simulink library "Simple_lib"  (R2018b)
settings: Solver=ode45  StartTime=0.0  StopTime=10.0  RelTol=1e-3  EnableMultiTasking=on
undefined symbols (not defined in the file or in its folder): Acceptance, beta, C, C_J, C_P, c_wall, dGain, DiscIntNeverNeededParam, Duplex, Electrical_lib, grab, h_fe, i, i3, K_T, Kman, KmanCE, mu_s, n_rev, R_arm, Simplex, systemTs, tau_0, TinIC, Ts, w_0, wallMass, Watch_lib
libraries: $bdroot x407, PlantUtilityBlockset_lib x30, peGeneralControl x22, simulink x11
(part 4 of 14)

== system Simple_lib/Magnetic ==
  BiGain : Subsystem  mask{k_level=-1, k_flow=-1}
      mask prompts: k_level "Level Gain"; k_flow "Flow Gain"
      settings: AttributesFormatString="%<k_flow>   %<k_level>"
      mask Display:
      | patch( [0 1 0],[1 0 -1])
      | plot( [0 -1 0],[1 0 -1])
  Core : Subsystem  mask{b=.5}
      mask prompts: b "Damping coefficient (Ns/m)"
      settings: AttributesFormatString=%<b> Ns/m
      mask Display:
      | plot([-1 1], [0.5 0.5])
      | plot([-1 1], [-0.5 -0.5])
      | 
      | color('white')
      | plot([-1 1 1 -1 -1], [-1 -1 1 1 -1])
  Core_old : Subsystem  mask{b=.9*sqrt(2e-1*3e-1)}
      mask prompts: b "Damping coefficient (Ns/m)"
      settings: AttributesFormatString=%<b> Ns/m
      mask Display:
      | plot([-1 1], [0.5 0.5])
      | plot([-1 1], [-0.5 -0.5])
      | 
      | color('white')
      | plot([-1 1 1 -1 -1], [-1 -1 1 1 -1])
  Friction : Subsystem  mask{grab=1, s=1, Ki=100}
      mask prompts: s "sigma"
      mask Display:
      | plot([0 .1],[1.7 1.7]);
      | plot([0 .1],[-1.7 -1.7]);
      | plot([.2 .3],[1.7 1.7]);
      | plot([.2 .3],[-1.7 -1.7]);
      | plot([.4 .5],[1.7 1.7]);
      | plot([.4 .5],[-1.7 -1.7]);
      | plot([.6 .7],[1.7 1.7]);
      | plot([.6 .7],[-1.7 -1.7]);
      | plot([.8 .9],[1.7 1.7]);
      | plot([.8 .9],[-1.7 -1.7]);
      | 
      | patch([0 1 1 0],[2 2 2.1 2.1]);
      | patch([0 1 1 0],[-2 -2 -2.1 -2.1]);
      | color('white');
      | plot([0 1],[3 3]);
      | plot([0 1],[-3 -3]);
  Sink : Subsystem  mask{m=0.01}
      mask prompts: m "Inertia (kg)"
      settings: AttributesFormatString=%<m> kg
      mask Display:
      | %color('white');
      | %plot([0 4],[1 1]);
      | %plot([0 4],[-1 -1]);
      | %color('black')
      | %plot([0 2],[0 0]);
      | plot([-1 -.9 -.8 0 .8 .9 1  .9  .8  0 -.8 -.9 -1],      [ 0  .9 .9 1 .9 .9 0 -.9 -.9 -1 -.9 -.9  0]);
  Source : Subsystem  mask{m=0.1, v_0=0}
      mask prompts: m "Inertia (kg)"; v_0 "Initial velocity (m/s)"
      settings: AttributesFormatString=%<m> kg
      mask Display:
      | %color('white');
      | %plot([-1 4],[1 1]);
      | %plot([-1 4],[-1 -1]);
      | %color('black')
      | %plot([1 4],[0 0]);
      | plot([-1 -.9 -.8 0 .8 .9 1  .9  .8  0 -.8 -.9 -1],      [ 0  .9 .9 1 .9 .9 0 -.9 -.9 -1 -.9 -.9  0]);
      | %plot([4 4.5 4.5 4],[0 -0.25 0.25 0])
  SpringDamper : Subsystem  mask{k_spring=1000, b_damper=0, b_spring=inf, m_out=0, m_split=0, v_0=0, s_0=0}
      mask prompts: k_spring "Stiffness (N/m)"; b_damper "Parallel Damping (Ns/m)"; b_spring "Series Damping (Ns/m)"; m_out "Output Inertia (kg)"; m_split "Split inertia (kg)"; v_0 "Initial speed (m/s)"; s_0 "Initial rotation (m)"
      mask Display:
      | %color('white')
      | %plot([-1 1 1 -1 -1], [-1 -1 1 1 -1])
      | %color('black')
      | %plot([1.0 1.18 1.18 1.0], [0 .2 -.2 0])
      | plot(-1+2*[-0.0625
      |    -0.0421
      |    -0.0129
      |     0.0230
      |     0.0625
      |     0.1020
      |     0.1379
      |     0.1671
      |     0.1875
      |     0.1984
      |     0.2004
      |     0.1958
      |     0.1875
      |     0.1792
      |     0.1746
      |     0.1766
      |     0.1875
      |     0.2079
      |     0.2371
      |     0.2730
      |     0.3125
      |     0.3520
      |     0.3879
      |     0.4171
      |     0.4375
      |     0.4484
      |     0.4504
      |     0.4458
      |     0.4375
      |     0.4292
      |     0.4246
      |     0.4266
      |     0.4375
      |     0.4579
      |     0.4871
      |     0.5230
      |     0.5625
      |     0.6020
      |     0.6379
      |     0.6671
      |     0.6875
      |     0.6984
      |     0.7004
      |     0.6958
      |     0.6875
      |     0.6792
      |     0.6746
      |     0.6766
      |     0.6875
      |     0.7079
      |     0.7371
      |     0.7730
      |     0.8125
      |     0.8520
      |     0.8879
      |     0.9171
      |     0.9375
      |     0.9484
      |     0.9504
      |     0.9458
      |     0.9375
      |     0.9292
      |     0.9246
      |     0.9266
      |     0.9375], [    0
      |     0.3827
      |     0.7071
      |     0.9239
      |     1.0000
      |     0.9239
      |     0.7071
      |     0.3827
      |     0.0000
      |    -0.3827
      |    -0.7071
      |    -0.9239
      |    -1.0000
      |    -0.9239
      |    -0.7071
      |    -0.3827
      |    -0.0000
      |     0.3827
      |     0.7071
      |     0.9239
      |     1.0000
      |     0.9239
      |     0.7071
      |     0.3827
      |     0.0000
      |    -0.3827
      |    -0.7071
      |    -0.9239
      |    -1.0000
      |    -0.9239
      |    -0.7071
      |    -0.3827
      |    -0.0000
      |     0.3827
      |     0.7071
      |     0.9239
      |     1.0000
      |     0.9239
      |     0.7071
      |     0.3827
      |     0.0000
      |    -0.3827
      |    -0.7071
      |    -0.9239
      |    -1.0000
      |    -0.9239
      |    -0.7071
      |    -0.3827
      |    -0.0000
      |     0.3827
      |     0.7071
      |     0.9239
      |     1.0000
      |     0.9239
      |     0.7071
      |     0.3827
      |     0.0000
      |    -0.3827
      |    -0.7071
      |    -0.9239
      |    -1.0000
      |    -0.9239
      |    -0.7071
      |    -0.3827
      |    -0.0000])
      | 
      | %color('black')
      | plot( [-1 0.3], [0 0]-3 )
      | plot( .3*[1 1],.9*[-1 1]-3 )
      | plot(  [0 1 1 0], [1 1 -1 -1]-3 )
      | %color('white')
      | %plot([-1 1], [1.1 1.1])
      | %plot([-1 1 1 -1 -1], [-1 -1 1 1 -1])
  Stiffness : Subsystem  mask{k_spring=1000, s_0=0, I_spring=0, b_series=inf}
      mask prompts: k_spring "Stiffness (N/m)"; s_0 "Initial displacement (m)"; I_spring "Inertia (kg)"; b_series "Series damping (Ns/m)"
      settings: AttributesFormatString=|
      | %<k_spring> N/m
      | %<s_0> m
      mask Display:
      | %color('black')
      | plot(   [    0     0.3827     0.7071     0.9239     1.0000     0.9239     0.7071     0.3827     0.0000    -0.3827    -0.7071    -0.9239    -1.0000    -0.9239    -0.7071    -0.3827    -0.0000     0.3827     0.7071     0.9239     1.0000     0.9239     0.7071     0.3827     0.0000    -0.3827    -0.7071    -0.9239    -1.0000    -0.9239    -0.7071    -0.3827    -0.0000     0.3827     0.7071     0.9239     1.0000     0.9239     0.7071     0.3827     0.0000    -0.3827    -0.7071    -0.9239    -1.0000    -0.9239    -0.7071    -0.3827    -0.0000     0.3827     0.7071     0.9239     1.0000     0.9239     0.7071     0.3827     0.0000    -0.3827    -0.7071    -0.9239    -1.0000    -0.9239    -0.7071    -0.3827    -0.0000],   -.5+[-0.0625    -0.0421    -0.0129     0.0230     0.0625     0.1020     0.1379     0.1671     0.1875     0.1984     0.2004     0.1958     0.1875     0.1792     0.1746     0.1766     0.1875     0.2079     0.2371     0.2730     0.3125     0.3520     0.3879     0.4171     0.4375     0.4484     0.4504     0.4458     0.4375     0.4292     0.4246     0.4266     0.4375     0.4579     0.4871     0.5230     0.5625     0.6020     0.6379     0.6671     0.6875     0.6984     0.7004     0.6958     0.6875     0.6792     0.6746     0.6766     0.6875     0.7079     0.7371     0.7730     0.8125     0.8520     0.8879     0.9171     0.9375     0.9484     0.9504     0.9458     0.9375     0.9292     0.9246     0.9266     0.9375])
      | color('white')
      | plot([-1 1 1 -1 -1], [-1 -1 1 1 -1])
  _in : Subsystem  InitFcn=""  mask{Level=MMF, Flow=Phi}
      mask prompts: Level "Level variable name:"; Flow "Flow variable name:"
      mask init:
      | init_in
      mask Display:
      | %% Icon for flow in
      | % Signally design
      | %plot([0 2 2 3], [1 1 0 0])
      | %plot([1 3 2 1 0 2], [0.6 0.6 0.4 0.6 0.4 0.4])
      | %patch([1 3 2],[0.6 0.6 0.4])
      | %plot([0 1 1], [1 1 0.6])
      | %plot([1 1 0], [0.4 -1 -1])
      | 
      | %color('white')
      | %plot([0 3], [2 2])
      | %plot([0 3], [-2 -2])
      | 
      | %% Bolder design
      | %patch( [0 1 -1], [0 1 1])
      | %plot( [-1 1], [1.051 1.05])
      | %patch( [-0.1 -0.1 -1], [0.95 0 0.95])
      | patch( [-0.1 -0.1 -1], [1 0 1])
      | patch( [0.1 0.1 1], [1 0 1])
      | plot( [0.1 1 -1 -0.1], [0 -2 -2 0]*0.5)
      | %patch( [-0.1 0.1 0.1 -0.1], [0 0 1 1], [1 1 1])
      | %patch( [-1 0.1 0.1 -1], [1 1 0.95 0.95], [1 1 1])
      | 
      | %% Size the box
      | color('white')
      | plot( [-1 1], [2 2])
      | plot( [-1 1], -[2 2])
  _out : Subsystem  Tag=Electrical  mask{Level=v, Flow=F}
      mask prompts: Level "Level variable name:"; Flow "Flow variable name:"
      mask init:
      | init_out
      mask Display:
      | % This is a new mask on top of the base mask.
      | % Use "View base mask" link below to see the base mask.
      | % Icon for flow out
      | %% Complex icon
      | %plot([0 1 1], [0 0 0.4])
      | %plot([1 1 3], [0.6 1 1])
      | %plot([1 3 2 1 0 2], [0.6 0.6 0.4 0.6 0.4 0.4])
      | %patch([0 2 1],[0.4 0.4 0.6])
      | %plot([3 2 2], [1 1 0.6])
      | %plot([2.2 2.2], [1 0.6])
      | %plot([1.8 1.8], [1 0.6])
      | %plot([1.6 2.4], [0 0])
      | %plot([2 2], [0.1 -0.1])
      | %plot([2 2], [0.4 0.2])
      | %plot([2 2 3], [-0.2 -1 -1])
      | 
      | %color('white')
      | %plot([0 3], [2 2])
      | %plot([0 3], [-2 -2])
      | 
      | %% Bolder icon
      | plot([-1 0 1], [0 -1 0])
      | %patch([-1 1 0 -1], [1 1 2 1]*1-1)
      | patch([-1 -.2 -.2], [0 0 1])
      | patch([1 .2 .2], [0 0 1])
      | %patch( [-0.1 0.1 0.1 -0.1], [0 0 1 1], [1 1 1])
      | plot(0.2*[-1 1],-0.3*[1  1]+0*1.5)
      | plot([0 0],[-0.15 -0.45]+0*1.5)
      | 
      | 
      | color('white')
      | plot( [-1 1], [2 2])
      | plot( [-1 1], -[2 2])
  magR : Subsystem  mask{b=.9*sqrt(2e-1*3e-1)}
      mask prompts: b "Damping coefficient (Ns/m)"
      settings: AttributesFormatString=%<b> Ns/m
      mask Display:
      | plot([-1 1], [0.5 0.5])
      | plot([-1 1], [-0.5 -0.5])
      | 
      | color('white')
      | plot([-1 1 1 -1 -1], [-1 -1 1 1 -1])

== system Simple_lib/Rotational ==
  BiGain : Subsystem  mask{k_level=1, k_flow=1}
      mask prompts: k_level "Potential Gain"; k_flow "Flow Gain"
      settings: AttributesFormatString="%<k_flow>   %<k_level>"
      mask Display:
      | patch( [0 1 0],[1 0 -1])
      | plot( [0 -1 0],[1 0 -1])
  Damping : Subsystem  mask{b=10}
      mask prompts: b "Damping coefficient (Nms/rad)"
      mask Display:
      | %color('black')
      | plot( [0 0],-[-1 0.3] )
      | plot( .9*[-1 -.8 .8 1 ],-.3*[ .6 1 1 .6] )
      | plot( [1 1 -1 -1],-[0 1 1 0] )
      | color('white')
      | %plot([-1 1], [1.1 1.1])
      | plot([-1 1 1 -1 -1]*1.1, [-1 -1 1 1 -1]*2)
  Friction : Subsystem  mask{grab=.03, s=.2, Ki=1}
      mask prompts: s "sigma"
      mask Display:
      | plot([0 .1],[1.7 1.7]);
      | plot([0 .1],[-1.7 -1.7]);
      | plot([.2 .3],[1.7 1.7]);
      | plot([.2 .3],[-1.7 -1.7]);
      | plot([.4 .5],[1.7 1.7]);
      | plot([.4 .5],[-1.7 -1.7]);
      | plot([.6 .7],[1.7 1.7]);
      | plot([.6 .7],[-1.7 -1.7]);
      | plot([.8 .9],[1.7 1.7]);
      | plot([.8 .9],[-1.7 -1.7]);
      | 
      | patch([0 1 1 0],[2 2 2.1 2.1]);
      | patch([0 1 1 0],[-2 -2 -2.1 -2.1]);
      | color('white');
      | plot([0 1],[3 3]);
      | plot([0 1],[-3 -3]);
  Inertia : Subsystem  mask{I=0.01}
      mask prompts: I "Inertia (kgm^2)"
      settings: AttributesFormatString=%<I> kgm2
      mask Display:
      | %color('white');
      | %plot([0 4],[1 1]);
      | %plot([0 4],[-1 -1]);
      | %color('black')
      | %plot([0 2],[0 0]);
      | plot([-1 -.9 -.5 0 .5 .9 1  .9  .5  0 -.5 -.9 -1]+3,      [ 0  .5 .9 1 .9 .5 0 -.5 -.9 -1 -.9 -.5  0]);
  Lump : Subsystem  mask{w_0=w_0, max_accel=inf, conserved_quantity_name=Momentum, energy_name=Energy}
      mask prompts: w_0 "Initial velocity (rad/s)"; max_accel "Max accel (m/s/s)"; conserved_quantity_name "Conserved quantity name"; energy_name "Energy name"
      mask init:
      | init_lump
      mask Display:
      | %color('white');
      | %plot([-1 4],[1 1]);
      | %plot([-1 4],[-1 -1]);
      | %color('black')
      | %plot([1 4],[0 0]);
      | plot([-1 -.9 -.5 0 .5 .9 1  .9  .5  0 -.5 -.9 -1],      [ 0  .5 .9 1 .9 .5 0 -.5 -.9 -1 -.9 -.5  0]);
      | %plot([4 4.5 4.5 4],[0 -0.25 0.25 0])
  M1 : Subsystem
      mask Display:
      | plot([-1 -.9 -.5 0 .5 .9 1  .9  .5  0 -.5 -.9 -1],      [ 0  .5 .9 1 .9 .5 0 -.5 -.9 -1 -.9 -.5  0]);
      | disp('M')
  NonLinear Compliance : Subsystem  mask{k_spring=0, theta_0=0, I_spring=0, b_series=inf}
      mask prompts: k_spring "Stiffness (Nm/rad)"; theta_0 "Initial displacement (rad)"; I_spring "Inertia (kgm^2)"; b_series "Series damping (Nms/rad)"
      mask Display:
      | %color('black')
      | plot(   [    0     0.3827     0.7071     0.9239     1.0000     0.9239     0.7071     0.3827     0.0000    -0.3827    -0.7071    -0.9239    -1.0000    -0.9239    -0.7071    -0.3827    -0.0000     0.3827     0.7071     0.9239     1.0000     0.9239     0.7071     0.3827     0.0000    -0.3827    -0.7071    -0.9239    -1.0000    -0.9239    -0.7071    -0.3827    -0.0000     0.3827     0.7071     0.9239     1.0000     0.9239     0.7071     0.3827     0.0000    -0.3827    -0.7071    -0.9239    -1.0000    -0.9239    -0.7071    -0.3827    -0.0000     0.3827     0.7071     0.9239     1.0000     0.9239     0.7071     0.3827     0.0000    -0.3827    -0.7071    -0.9239    -1.0000    -0.9239    -0.7071    -0.3827    -0.0000],   -.5+[-0.0625    -0.0421    -0.0129     0.0230     0.0625     0.1020     0.1379     0.1671     0.1875     0.1984     0.2004     0.1958     0.1875     0.1792     0.1746     0.1766     0.1875     0.2079     0.2371     0.2730     0.3125     0.3520     0.3879     0.4171     0.4375     0.4484     0.4504     0.4458     0.4375     0.4292     0.4246     0.4266     0.4375     0.4579     0.4871     0.5230     0.5625     0.6020     0.6379     0.6671     0.6875     0.6984     0.7004     0.6958     0.6875     0.6792     0.6746     0.6766     0.6875     0.7079     0.7371     0.7730     0.8125     0.8520     0.8879     0.9171     0.9375     0.9484     0.9504     0.9458     0.9375     0.9292     0.9246     0.9266     0.9375])
      | color('white')
      | plot([-1 1 1 -1 -1], [-1 -1 1 1 -1])
  Power : Subsystem
      mask Display:
      | plot([-1 -.9 -.5 0 .5 .9 1  .9  .5  0 -.5 -.9 -1],      [ 0  .5 .9 1 .9 .5 0 -.5 -.9 -1 -.9 -.5  0]);
      | disp('P')
  Speed : Subsystem
      mask Display:
      | plot([0.8 1 0.8 0.8]*0.5,[-1 0 1 -1])
      | 
      | color('black')
      | plot([-1 1]*0.5,[0 0])
      | %plot([1 1.2 1]*0.5-0.2,[-1 0 1])
      | 
      | %color('white')
      | %plot([-1 1],[-1 -1])
      | %plot([-1 1],[1 1])
  SpringDamper : Subsystem  mask{k_spring=1, b_damper=0, b_spring=inf, I_out=0, I_split=0, w_0=0, theta_0=0}
      mask prompts: k_spring "Stiffness (Nm/rad)"; b_damper "Parallel Damping (Nms/rad)"; b_spring "Series Damping (Nms/rad)"; I_out "Output Inertia (kgm^2)"; I_split "Split inertia (kgm^2)"; w_0 "Initial speed (rad/s)"; theta_0 "Initial rotation (rad)"
      mask Display:
      | %color('white')
      | %plot([-1 1 1 -1 -1], [-1 -1 1 1 -1])
      | %color('black')
      | %plot([1.0 1.18 1.18 1.0], [0 .2 -.2 0])
      | plot(-1+2*[-0.0625
      |    -0.0421
      |    -0.0129
      |     0.0230
      |     0.0625
      |     0.1020
      |     0.1379
      |     0.1671
      |     0.1875
      |     0.1984
      |     0.2004
      |     0.1958
      |     0.1875
      |     0.1792
      |     0.1746
      |     0.1766
      |     0.1875
      |     0.2079
      |     0.2371
      |     0.2730
      |     0.3125
      |     0.3520
      |     0.3879
      |     0.4171
      |     0.4375
      |     0.4484
      |     0.4504
      |     0.4458
      |     0.4375
      |     0.4292
      |     0.4246
      |     0.4266
      |     0.4375
      |     0.4579
      |     0.4871
      |     0.5230
      |     0.5625
      |     0.6020
      |     0.6379
      |     0.6671
      |     0.6875
      |     0.6984
      |     0.7004
      |     0.6958
      |     0.6875
      |     0.6792
      |     0.6746
      |     0.6766
      |     0.6875
      |     0.7079
      |     0.7371
      |     0.7730
      |     0.8125
      |     0.8520
      |     0.8879
      |     0.9171
      |     0.9375
      |     0.9484
      |     0.9504
      |     0.9458
      |     0.9375
      |     0.9292
      |     0.9246
      |     0.9266
      |     0.9375], [    0
      |     0.3827
      |     0.7071
      |     0.9239
      |     1.0000
      |     0.9239
      |     0.7071
      |     0.3827
      |     0.0000
      |    -0.3827
      |    -0.7071
      |    -0.9239
      |    -1.0000
      |    -0.9239
      |    -0.7071
      |    -0.3827
      |    -0.0000
      |     0.3827
      |     0.7071
      |     0.9239
      |     1.0000
      |     0.9239
      |     0.7071
      |     0.3827
      |     0.0000
      |    -0.3827
      |    -0.7071
      |    -0.9239
      |    -1.0000
      |    -0.9239
      |    -0.7071
      |    -0.3827
      |    -0.0000
      |     0.3827
      |     0.7071
      |     0.9239
      |     1.0000
      |     0.9239
      |     0.7071
      |     0.3827
      |     0.0000
      |    -0.3827
      |    -0.7071
      |    -0.9239
      |    -1.0000
      |    -0.9239
      |    -0.7071
      |    -0.3827
      |    -0.0000
      |     0.3827
      |     0.7071
      |     0.9239
      |     1.0000
      |     0.9239
      |     0.7071
      |     0.3827
      |     0.0000
      |    -0.3827
      |    -0.7071
      |    -0.9239
      |    -1.0000
      |    -0.9239
      |    -0.7071
      |    -0.3827
      |    -0.0000])
      | 
      | %color('black')
      | plot( [-1 0.3], [0 0]-3 )
      | plot( .3*[1 1],.9*[-1 1]-3 )
      | plot(  [0 1 1 0], [1 1 -1 -1]-3 )
      | %color('white')
      | %plot([-1 1], [1.1 1.1])
      | %plot([-1 1 1 -1 -1], [-1 -1 1 1 -1])
  Stiffness : Subsystem  mask{k_spring=1e4, theta_0=0, I_spring=0, b_series=1}
      mask prompts: k_spring "Stiffness (Nm/rad)"; theta_0 "Initial displacement (rad)"; I_spring "Inertia (kgm^2)"; b_series "Series damping (Nms/rad)"
      mask Display:
      | %color('black')
      | plot(   [    0     0.3827     0.7071     0.9239     1.0000     0.9239     0.7071     0.3827     0.0000    -0.3827    -0.7071    -0.9239    -1.0000    -0.9239    -0.7071    -0.3827    -0.0000     0.3827     0.7071     0.9239     1.0000     0.9239     0.7071     0.3827     0.0000    -0.3827    -0.7071    -0.9239    -1.0000    -0.9239    -0.7071    -0.3827    -0.0000     0.3827     0.7071     0.9239     1.0000     0.9239     0.7071     0.3827     0.0000    -0.3827    -0.7071    -0.9239    -1.0000    -0.9239    -0.7071    -0.3827    -0.0000     0.3827     0.7071     0.9239     1.0000     0.9239     0.7071     0.3827     0.0000    -0.3827    -0.7071    -0.9239    -1.0000    -0.9239    -0.7071    -0.3827    -0.0000],   -.5+[-0.0625    -0.0421    -0.0129     0.0230     0.0625     0.1020     0.1379     0.1671     0.1875     0.1984     0.2004     0.1958     0.1875     0.1792     0.1746     0.1766     0.1875     0.2079     0.2371     0.2730     0.3125     0.3520     0.3879     0.4171     0.4375     0.4484     0.4504     0.4458     0.4375     0.4292     0.4246     0.4266     0.4375     0.4579     0.4871     0.5230     0.5625     0.6020     0.6379     0.6671     0.6875     0.6984     0.7004     0.6958     0.6875     0.6792     0.6746     0.6766     0.6875     0.7079     0.7371     0.7730     0.8125     0.8520     0.8879     0.9171     0.9375     0.9484     0.9504     0.9458     0.9375     0.9292     0.9246     0.9266     0.9375])
      | color('white')
      | plot([-1 1 1 -1 -1], [-1 -1 1 1 -1])
  Torque : Subsystem
      mask Display:
      | plot([-1 0 1],[0.8 1 0.8]*0.5)
      | plot([-1 0 1],[1 1.2 1]*0.5-0.2)
      | 
      | color('black')
      | plot([0 0],[-1 1]*0.5)
      | 
      | color('white')
      | plot([-1 1],[-1 -1])
      | plot([-1 1],[1 1])
  _in : Subsystem  InitFcn=""  mask{Level=w, Flow=tau}
      mask prompts: Level "Level variable name:"; Flow "Flow variable name:"
      mask init:
      | init_in
      mask Display:
      | %% Icon for flow in
      | % Signally design
      | %plot([0 2 2 3], [1 1 0 0])
      | %plot([1 3 2 1 0 2], [0.6 0.6 0.4 0.6 0.4 0.4])
      | %patch([1 3 2],[0.6 0.6 0.4])
      | %plot([0 1 1], [1 1 0.6])
      | %plot([1 1 0], [0.4 -1 -1])
      | 
      | %color('white')
      | %plot([0 3], [2 2])
      | %plot([0 3], [-2 -2])
      | 
      | %% Bolder design
      | %patch( [0 1 -1], [0 1 1])
      | %plot( [-1 1], [1.051 1.05])
      | %patch( [-0.1 -0.1 -1], [0.95 0 0.95])
      | patch( [-0.1 -0.1 -1], [1 0 1])
      | patch( [0.1 0.1 1], [1 0 1])
      | plot( [0.1 1 -1 -0.1], [0 -2 -2 0]*0.5)
      | %patch( [-0.1 0.1 0.1 -0.1], [0 0 1 1], [1 1 1])
      | %patch( [-1 0.1 0.1 -1], [1 1 0.95 0.95], [1 1 1])
      | 
      | %% Size the box
      | color('white')
      | plot( [-1 1], [2 2])
      | plot( [-1 1], -[2 2])
  _out : Subsystem  Tag=Electrical  mask{Level=w, Flow=tau}
      mask prompts: Level "Level variable name:"; Flow "Flow variable name:"
      mask init:
      | init_out
      mask Display:
      | % This is a new mask on top of the base mask.
      | % Use "View base mask" link below to see the base mask.
      | % Icon for flow out
      | %% Complex icon
      | %plot([0 1 1], [0 0 0.4])
      | %plot([1 1 3], [0.6 1 1])
      | %plot([1 3 2 1 0 2], [0.6 0.6 0.4 0.6 0.4 0.4])
      | %patch([0 2 1],[0.4 0.4 0.6])
      | %plot([3 2 2], [1 1 0.6])
      | %plot([2.2 2.2], [1 0.6])
      | %plot([1.8 1.8], [1 0.6])
      | %plot([1.6 2.4], [0 0])
      | %plot([2 2], [0.1 -0.1])
      | %plot([2 2], [0.4 0.2])
      | %plot([2 2 3], [-0.2 -1 -1])
      | 
      | %color('white')
      | %plot([0 3], [2 2])
      | %plot([0 3], [-2 -2])
      | 
      | %% Bolder icon
      | plot([-1 0 1], [0 -1 0])
      | %patch([-1 1 0 -1], [1 1 2 1]*1-1)
      | patch([-1 -.2 -.2], [0 0 1])
      | patch([1 .2 .2], [0 0 1])
      | %patch( [-0.1 0.1 0.1 -0.1], [0 0 1 1], [1 1 1])
      | plot(0.2*[-1 1],-0.3*[1  1]+0*1.5)
      | plot([0 0],[-0.15 -0.45]+0*1.5)
      | 
      | 
      | color('white')
      | plot( [-1 1], [2 2])
      | plot( [-1 1], -[2 2])

== system Simple_lib/Thermal ==
  CinWall : Subsystem  AncestorBlock=PlantUtilityBlockset_lib/Electrical/C0
      mask Display:
      | color('white')
      | plot([-1 1 1 -1 -1], [-1 -1 1 1 -1])
      | 
      | color('red')
      | plot([1.0 1.18 1.18 1.0], [0 .15 -.15 0])
      | patch([1.0 1.0 0.8 0.8 0.7 -0.9 -1.0 -1.0 -0.9  0.7  0.8 0.8   1.0 1.0],        [0.0 0.3 0.2 0.9 1.0 1.0   0.9 -0.9 -1.0 -1.0 -0.9 -0.2 -0.3 0.0],       [.8 0 0])
  R13 : Subsystem  AncestorBlock=PlantUtilityBlockset_lib/Electrical/R  mask{R=1/wallArea/h_A_W}
      mask prompts: R "Resistance"
      mask Display:
      | color('white')
      | plot([-1 1 1 -1 -1], [-1 -1 1 1 -1])
      | color('red')
      | plot([1.0 1.18 1.18 1.0], [0 .2 -.2 0])
      | plot([1 1],[-1 1])
      | plot([-8:8]/8, cos([-8:8])/2)
  R17 : Subsystem  AncestorBlock=PlantUtilityBlockset_lib/Electrical/R1  mask{R=LWall/kWall/wallArea/2}
      mask prompts: R "Resistance"
      mask Display:
      | color('white')
      | plot([-1 1 1 -1 -1], [-1 -1 1 1 -1])
      | color('red')
      | patch( [ -1 1 1 -1 -1],[-.51 -.51  -.49 -.49 -.51],[0.85 0 0])
      | patch( [ -1 1 1 -1 -1],[ .51  .51   .49  .49  .51],[0.85 0 0])
      | plot( [ .6 1],[-.5 .2])
      | plot( [ .3 .8],[-.5 .5])
      | plot( [ .0 .5],[-.5 .5])
      | plot( [-.3 .2],[-.5 .5])
      | plot( [-.6 -.1],[-.5 .5])
      | plot( [-.9 -.4],[-.5 .5])
      | plot( [-1 -.7],[-.1 .5])
      | %plot( [ -1 0 1 0 -1 0 1 0 -1 0 1 0 -1],[-6:6]/12)
  ThermoMeter : Subsystem
      mask Display:
      | color('white')
      | plot([-1 1 1 -1 -1], [-1 -1 1 1 -1])
      | color('black')
      | 
      | plot([-1 -.9 -.5 0 .5 .9 1  .9  .5  0 -.5 -.9 -1], ...
      |     [ 0  .5 .9 1 .9 .5 0 -.5 -.9 -1 -.9 -.5  0]);
      | plot(.7*[-1 1], .7*[-1 1])
      | plot(.7*[-1 1], .7*[1 -1])
      | 
      | %text(0, 0, 'p')

== system Simple_lib/Translational ==
  BiGain : Subsystem  mask{k_level=-1, k_flow=-1}
      mask prompts: k_level "Level Gain"; k_flow "Flow Gain"
      settings: AttributesFormatString="%<k_flow>   %<k_level>"
      mask Display:
      | patch( [0 1 0],[1 0 -1])
      | plot( [0 -1 0],[1 0 -1])
  Damping : Subsystem  mask{b=1}
      mask prompts: b "Damping coefficient (Ns/m)"
      settings: AttributesFormatString=%<b> Ns/m
      mask Display:
      | %color('black')
      | plot( [0 0],-[-1 0.3] )
      | plot( .9*[-1 -.8 .8 1 ],-.3*[ .6 1 1 .6] )
      | plot( [1 1 -1 -1],-[0 1 1 0] )
      | color('white')
      | %plot([-1 1], [1.1 1.1])
      | plot([-1 1 1 -1 -1]*1.1, [-1 -1 1 1 -1]*2)
  Friction : Subsystem  mask{grab=1, s=1, Ki=100}
      mask prompts: s "sigma"
      mask Display:
      | plot([0 .1],[1.7 1.7]);
      | plot([0 .1],[-1.7 -1.7]);
      | plot([.2 .3],[1.7 1.7]);
      | plot([.2 .3],[-1.7 -1.7]);
      | plot([.4 .5],[1.7 1.7]);
      | plot([.4 .5],[-1.7 -1.7]);
      | plot([.6 .7],[1.7 1.7]);
      | plot([.6 .7],[-1.7 -1.7]);
      | plot([.8 .9],[1.7 1.7]);
      | plot([.8 .9],[-1.7 -1.7]);
      | 
      | patch([0 1 1 0],[2 2 2.1 2.1]);
      | patch([0 1 1 0],[-2 -2 -2.1 -2.1]);
      | color('white');
      | plot([0 1],[3 3]);
      | plot([0 1],[-3 -3]);
  Sink : Subsystem  mask{m=0.01}
      mask prompts: m "Inertia (kg)"
      settings: AttributesFormatString=%<m> kg
      mask Display:
      | %color('white');
      | %plot([0 4],[1 1]);
      | %plot([0 4],[-1 -1]);
      | %color('black')
      | %plot([0 2],[0 0]);
      | plot([-1 -.9 -.8 0 .8 .9 1  .9  .8  0 -.8 -.9 -1],      [ 0  .9 .9 1 .9 .9 0 -.9 -.9 -1 -.9 -.9  0]);
  Source : Subsystem  mask{m=0.1, v_0=0}
      mask prompts: m "Inertia (kg)"; v_0 "Initial velocity (m/s)"
      settings: AttributesFormatString=%<m> kg
      mask Display:
      | %color('white');
      | %plot([-1 4],[1 1]);
      | %plot([-1 4],[-1 -1]);
      | %color('black')
      | %plot([1 4],[0 0]);
      | plot([-1 -.9 -.8 0 .8 .9 1  .9  .8  0 -.8 -.9 -1],      [ 0  .9 .9 1 .9 .9 0 -.9 -.9 -1 -.9 -.9  0]);
      | %plot([4 4.5 4.5 4],[0 -0.25 0.25 0])
  SpringDamper : Subsystem  mask{k_spring=1000, b_damper=0, b_spring=inf, m_out=0, m_split=0, v_0=0, s_0=0}
      mask prompts: k_spring "Stiffness (N/m)"; b_damper "Parallel Damping (Ns/m)"; b_spring "Series Damping (Ns/m)"; m_out "Output Inertia (kg)"; m_split "Split inertia (kg)"; v_0 "Initial speed (m/s)"; s_0 "Initial rotation (m)"
      mask Display:
      | %color('white')
      | %plot([-1 1 1 -1 -1], [-1 -1 1 1 -1])
      | %color('black')
      | %plot([1.0 1.18 1.18 1.0], [0 .2 -.2 0])
      | plot(-1+2*[-0.0625
      |    -0.0421
      |    -0.0129
      |     0.0230
      |     0.0625
      |     0.1020
      |     0.1379
      |     0.1671
      |     0.1875
      |     0.1984
      |     0.2004
      |     0.1958
      |     0.1875
      |     0.1792
      |     0.1746
      |     0.1766
      |     0.1875
      |     0.2079
      |     0.2371
      |     0.2730
      |     0.3125
      |     0.3520
      |     0.3879
      |     0.4171
      |     0.4375
      |     0.4484
      |     0.4504
      |     0.4458
      |     0.4375
      |     0.4292
      |     0.4246
      |     0.4266
      |     0.4375
      |     0.4579
      |     0.4871
      |     0.5230
      |     0.5625
      |     0.6020
      |     0.6379
      |     0.6671
      |     0.6875
      |     0.6984
      |     0.7004
      |     0.6958
      |     0.6875
      |     0.6792
      |     0.6746
      |     0.6766
      |     0.6875
      |     0.7079
      |     0.7371
      |     0.7730
      |     0.8125
      |     0.8520
      |     0.8879
      |     0.9171
      |     0.9375
      |     0.9484
      |     0.9504
      |     0.9458
      |     0.9375
      |     0.9292
      |     0.9246
      |     0.9266
      |     0.9375], [    0
      |     0.3827
      |     0.7071
      |     0.9239
      |     1.0000
      |     0.9239
      |     0.7071
      |     0.3827
      |     0.0000
      |    -0.3827
      |    -0.7071
      |    -0.9239
      |    -1.0000
      |    -0.9239
      |    -0.7071
      |    -0.3827
      |    -0.0000
      |     0.3827
      |     0.7071
      |     0.9239
      |     1.0000
      |     0.9239
      |     0.7071
      |     0.3827
      |     0.0000
      |    -0.3827
      |    -0.7071
      |    -0.9239
      |    -1.0000
      |    -0.9239
      |    -0.7071
      |    -0.3827
      |    -0.0000
      |     0.3827
      |     0.7071
      |     0.9239
      |     1.0000
      |     0.9239
      |     0.7071
      |     0.3827
      |     0.0000
      |    -0.3827
      |    -0.7071
      |    -0.9239
      |    -1.0000
      |    -0.9239
      |    -0.7071
      |    -0.3827
      |    -0.0000
      |     0.3827
      |     0.7071
      |     0.9239
      |     1.0000
      |     0.9239
      |     0.7071
      |     0.3827
      |     0.0000
      |    -0.3827
      |    -0.7071
      |    -0.9239
      |    -1.0000
      |    -0.9239
      |    -0.7071
      |    -0.3827
      |    -0.0000])
      | 
      | %color('black')
      | plot( [-1 0.3], [0 0]-3 )
      | plot( .3*[1 1],.9*[-1 1]-3 )
      | plot(  [0 1 1 0], [1 1 -1 -1]-3 )
      | %color('white')
      | %plot([-1 1], [1.1 1.1])
      | %plot([-1 1 1 -1 -1], [-1 -1 1 1 -1])
  Stiffness : Subsystem  mask{k_spring=1000, s_0=0, I_spring=0, b_series=inf}
      mask prompts: k_spring "Stiffness (N/m)"; s_0 "Initial displacement (m)"; I_spring "Inertia (kg)"; b_series "Series damping (Ns/m)"
      settings: AttributesFormatString=|
      | %<k_spring> N/m
      | %<s_0> m
      mask Display:
      | %color('black')
      | plot(   [    0     0.3827     0.7071     0.9239     1.0000     0.9239     0.7071     0.3827     0.0000    -0.3827    -0.7071    -0.9239    -1.0000    -0.9239    -0.7071    -0.3827    -0.0000     0.3827     0.7071     0.9239     1.0000     0.9239     0.7071     0.3827     0.0000    -0.3827    -0.7071    -0.9239    -1.0000    -0.9239    -0.7071    -0.3827    -0.0000     0.3827     0.7071     0.9239     1.0000     0.9239     0.7071     0.3827     0.0000    -0.3827    -0.7071    -0.9239    -1.0000    -0.9239    -0.7071    -0.3827    -0.0000     0.3827     0.7071     0.9239     1.0000     0.9239     0.7071     0.3827     0.0000    -0.3827    -0.7071    -0.9239    -1.0000    -0.9239    -0.7071    -0.3827    -0.0000],   -.5+[-0.0625    -0.0421    -0.0129     0.0230     0.0625     0.1020     0.1379     0.1671     0.1875     0.1984     0.2004     0.1958     0.1875     0.1792     0.1746     0.1766     0.1875     0.2079     0.2371     0.2730     0.3125     0.3520     0.3879     0.4171     0.4375     0.4484     0.4504     0.4458     0.4375     0.4292     0.4246     0.4266     0.4375     0.4579     0.4871     0.5230     0.5625     0.6020     0.6379     0.6671     0.6875     0.6984     0.7004     0.6958     0.6875     0.6792     0.6746     0.6766     0.6875     0.7079     0.7371     0.7730     0.8125     0.8520     0.8879     0.9171     0.9375     0.9484     0.9504     0.9458     0.9375     0.9292     0.9246     0.9266     0.9375])
      | color('white')
      | plot([-1 1 1 -1 -1], [-1 -1 1 1 -1])
  _in : Subsystem  InitFcn=""  mask{Level=v, Flow=F}
      mask prompts: Level "Level variable name:"; Flow "Flow variable name:"
      mask init:
      | init_in
      mask Display:
      | %% Icon for flow in
      | % Signally design
      | %plot([0 2 2 3], [1 1 0 0])
      | %plot([1 3 2 1 0 2], [0.6 0.6 0.4 0.6 0.4 0.4])
      | %patch([1 3 2],[0.6 0.6 0.4])
      | %plot([0 1 1], [1 1 0.6])
      | %plot([1 1 0], [0.4 -1 -1])
      | 
      | %color('white')
      | %plot([0 3], [2 2])
      | %plot([0 3], [-2 -2])
      | 
      | %% Bolder design
      | %patch( [0 1 -1], [0 1 1])
      | %plot( [-1 1], [1.051 1.05])
      | %patch( [-0.1 -0.1 -1], [0.95 0 0.95])
      | patch( [-0.1 -0.1 -1], [1 0 1])
      | patch( [0.1 0.1 1], [1 0 1])
      | plot( [0.1 1 -1 -0.1], [0 -2 -2 0]*0.5)
      | %patch( [-0.1 0.1 0.1 -0.1], [0 0 1 1], [1 1 1])
      | %patch( [-1 0.1 0.1 -1], [1 1 0.95 0.95], [1 1 1])
      | 
      | %% Size the box
      | color('white')
      | plot( [-1 1], [2 2])
      | plot( [-1 1], -[2 2])
  _out : Subsystem  Tag=Electrical  mask{Level=v, Flow=F}
      mask prompts: Level "Level variable name:"; Flow "Flow variable name:"
      mask init:
      | init_out
      mask Display:
      | % This is a new mask on top of the base mask.
      | % Use "View base mask" link below to see the base mask.
      | % Icon for flow out
      | %% Complex icon
      | %plot([0 1 1], [0 0 0.4])
      | %plot([1 1 3], [0.6 1 1])
      | %plot([1 3 2 1 0 2], [0.6 0.6 0.4 0.6 0.4 0.4])
      | %patch([0 2 1],[0.4 0.4 0.6])
      | %plot([3 2 2], [1 1 0.6])
      | %plot([2.2 2.2], [1 0.6])
      | %plot([1.8 1.8], [1 0.6])
      | %plot([1.6 2.4], [0 0])
      | %plot([2 2], [0.1 -0.1])
      | %plot([2 2], [0.4 0.2])
      | %plot([2 2 3], [-0.2 -1 -1])
      | 
      | %color('white')
      | %plot([0 3], [2 2])
      | %plot([0 3], [-2 -2])
      | 
      | %% Bolder icon
      | plot([-1 0 1], [0 -1 0])
      | %patch([-1 1 0 -1], [1 1 2 1]*1-1)
      | patch([-1 -.2 -.2], [0 0 1])
      | patch([1 .2 .2], [0 0 1])
      | %patch( [-0.1 0.1 0.1 -0.1], [0 0 1 1], [1 1 1])
      | plot(0.2*[-1 1],-0.3*[1  1]+0*1.5)
      | plot([0 0],[-0.15 -0.45]+0*1.5)
      | 
      | 
      | color('white')
      | plot( [-1 1], [2 2])
      | plot( [-1 1], -[2 2])

== system Simple_lib/Utility ==
  note: Experimenting with different graphical design for the Inflow and Outflow blocks.
  BiGain : Subsystem  mask{k_pot=0, k_flow=0}
      mask prompts: k_pot "Potential Gain"; k_flow "Flow Gain"
      mask Display:
      | %patch( [1 1.05 1.05 1],[-1 -1 1 1])
      | patch( [1 0 0],[0 1 -1])
      | plot( [0 1 1],[1 2 0])
  Bus Creator : BusCreator  Inputs=2
  Duplex : Subsystem  Tag=Electrical  Commented=on  InitFcn=initDuplex
      mask Display:
      | color('white')
      | plot([0 3], [2 2])
      | plot([0 3], [-2 -2])
      | color('black')
      | 
      | plot([0 1 1], [0 0 0.4])
      | plot([1 1 3], [0.6 1 1])
      | plot([1 3 2 1 0 2], [0.6 0.6 0.4 0.6 0.4 0.4])
      | patch([0 2 1],[0.4 0.4 0.6],[0,0,0])
      | plot([3 2 2], [1 1 0.6])
      | plot([2 2 3], [0.4 -1 -1])
  DuplexSav : Subsystem  Tag=Electrical  Commented=on  InitFcn=initDuplex
      mask Display:
      | plot([0 1 1], [0 0 0.4])
      | plot([1 1 3], [0.6 1 1])
      | plot([1 3 2 1 0 2], [0.6 0.6 0.4 0.6 0.4 0.4])
      | patch([0 2 1],[0.4 0.4 0.6],[0,0,0])
      | plot([3 2 2], [1 1 0.6])
      | plot([2.2 2.2], [1 0.6])
      | plot([1.8 1.8], [1 0.6])
      | plot([1.6 2.4], [0 0])
      | plot([2 2], [0.1 -0.1])
      | plot([2 2], [0.4 0.2])
      | plot([2 2 3], [-0.2 -1 -1])
      | 
      | color('white')
      | plot([0 3], [2 2])
      | plot([0 3], [-2 -2])
  Inflow : Subsystem  InitFcn=""
      mask init:
      | initInflow
      mask Display:
      | %% Icon for flow in
      | % Signally design
      | %plot([0 2 2 3], [1 1 0 0])
      | %plot([1 3 2 1 0 2], [0.6 0.6 0.4 0.6 0.4 0.4])
      | %patch([1 3 2],[0.6 0.6 0.4])
      | %plot([0 1 1], [1 1 0.6])
      | %plot([1 1 0], [0.4 -1 -1])
      | 
      | %color('white')
      | %plot([0 3], [2 2])
      | %plot([0 3], [-2 -2])
      | 
      | %% Bolder design
      | %patch( [0 1 -1], [0 1 1])
      | %plot( [-1 1], [1.051 1.05])
      | %patch( [-0.1 -0.1 -1], [0.95 0 0.95])
      | patch( [-0.1 -0.1 -1], [1 0 1])
      | patch( [0.1 0.1 1], [1 0 1])
      | plot( [0.1 1 -1 -0.1], [0 -2 -2 0]*0.5)
      | %patch( [-0.1 0.1 0.1 -0.1], [0 0 1 1], [1 1 1])
      | %patch( [-1 0.1 0.1 -1], [1 1 0.95 0.95], [1 1 1])
      | 
      | %% Size the box
      | color('white')
      | plot( [-1 1], [2 2])
      | plot( [-1 1], -[2 2])
  Inflow_old : Subsystem  InitFcn=""
      mask init:
      | initInput
      mask Display:
      | %% Plot upstream flow
      | %patch( [0 1 -1 0], [0 2 2 0])
      | %plot( [0 1 -1 0], [0 -2 -2 0])
      | %plot( [-1 -1], [-1 0])
      | 
      | %patch( [-1 0 0 1 1 -1 -1], [1 1 -1 -1 2 2 1])
      | %patch( [0 1 -1 0], [0 2 2 0])
      | 
      | 
      | patch( [-1 1 1 0 0 -1], [2 2 -1 -1 1 1])
      | plot( [-1 -1 0 0], [1 -2 -2 -1])
  Inflow_old1 : Subsystem  InitFcn=""
      mask init:
      | initInput
      mask Display:
      | %% Plot upstream flow
      | %patch( [0 1 -1 0], [0 2 2 0])
      | %plot( [0 1 -1 0], [0 -2 -2 0])
      | %plot( [-1 -1], [-1 0])
      | 
      | %patch( [-1 0 0 1 1 -1 -1], [1 1 -1 -1 2 2 1])
      | %patch( [0 1 -1 0], [0 2 2 0])
      | 
      | 
      | %patch( [-1 1 1 0 0 -1], [2 2 -1 -1 1 1])
      | %plot( [-1 -1 0 0], [1 -2 -2 -1])
      | 
      | plot([-1 -1],[-2 2])
      | %plot([0 0],[-1 1])
      | %patch([0 1 1 0], [-.25 -0.25 1 1])
      | patch(.4*[0 1 1 0], [0 0 2 2])
      | %plot(0.9*[1 1],[0 2])
      | 
      | %color('white')
      | %plot([-1 1],[-2 -2])
      | %plot([-1 1],[2 2])
  Mux : Mux  Inputs=2
  Outflow : Subsystem  Tag=Electrical
      mask init:
      | initOutflow
      mask Display:
      | % This is a new mask on top of the base mask.
      | % Use "View base mask" link below to see the base mask.
      | % Icon for flow out
      | %% Complex icon
      | %plot([0 1 1], [0 0 0.4])
      | %plot([1 1 3], [0.6 1 1])
      | %plot([1 3 2 1 0 2], [0.6 0.6 0.4 0.6 0.4 0.4])
      | %patch([0 2 1],[0.4 0.4 0.6])
      | %plot([3 2 2], [1 1 0.6])
      | %plot([2.2 2.2], [1 0.6])
      | %plot([1.8 1.8], [1 0.6])
      | %plot([1.6 2.4], [0 0])
      | %plot([2 2], [0.1 -0.1])
      | %plot([2 2], [0.4 0.2])
      | %plot([2 2 3], [-0.2 -1 -1])
      | 
      | %color('white')
      | %plot([0 3], [2 2])
      | %plot([0 3], [-2 -2])
      | 
      | %% Bolder icon
      | plot([-1 0 1], [0 -1 0])
      | %patch([-1 1 0 -1], [1 1 2 1]*1-1)
      | patch([-1 -.2 -.2], [0 0 1])
      | patch([1 .2 .2], [0 0 1])
      | %patch( [-0.1 0.1 0.1 -0.1], [0 0 1 1], [1 1 1])
      | 
      | % cross
      | %plot(0.2*[-1 1],-0.3*[1  1]+0*1.5)
      | %plot([0 0],[-0.15 -0.45]+0*1.5)
      | % fan
      | plot([-0.2 0],[0 -1])
      | %plot([-0.4 0],[0 -1])
      | plot([-0.6 0],[0 -1])
      | %plot([-0.8 0],[0 -1])
      | %plot([0 0],[0 -1])
      | plot([0.2 0],[0 -1])
      | %plot([0.4 0],[0 -1])
      | plot([0.6 0],[0 -1])
      | %plot([0.8 0],[0 -1])
      | color('white')
      | plot( [-1 1], [2 2])
      | plot( [-1 1], -[2 2])
  Outflow_old : Subsystem  Tag=Electrical
      mask Display:
      | %plot([-1 1 0 -1], [1 1 0 1]*2-2)
      | %patch([-1 1 0 -1], [1 1 2 1]*2-2)
      | 
      | patch( [1 -1 -1 0 0 1], [2 2 -1 -1 1 1])
      | plot( [1 1 0 0], [1 -2 -2 -1])
      | plot([1 1 2]/2, [1 -1 -1])
      | %plot([1 .6 .6 1], [1  1 -1 -1]*.6)
      | %plot([1 .3 .3 1], [1  1 -1 -1]*1.3)
      | plot([1 .75 .75 1], [1  1 -1 -1]*.6)
      | plot([1 .25 .25 1], [1  1 -1 -1]*1.45)
  Outflow_old1 : Subsystem  Tag=Electrical
      mask Display:
      | plot([1 1],[-1 1])
      | patch([0 1 1 0]-1, [0 0 1 1])
      | 
      | color('white')
      | %plot([-1 1],[-2 -2])
      | %plot([-1 1],[2 2])
  Pull : Subsystem  Tag=Electrical  Commented=on  InitFcn=initDuplex
      mask Display:
      | color('white')
      | plot([0 3], [2 2])
      | plot([0 3], [-2 -2])
      | color('black')
      | 
      | plot([0 1 1], [0 0 0.4])
      | plot([1 1 3], [0.6 1 1])
      | plot([1 3 2 1 0 2], [0.6 0.6 0.4 0.6 0.4 0.4])
      | patch([0 2 1],[0.4 0.4 0.6],[0,0,0])
      | plot([3 2 2], [1 1 0.6])
      | plot([2 2 3], [0.4 -1 -1])
  Push : Subsystem  Commented=on  InitFcn=initSimplex
      mask Display:
      | color('white')
      | plot([0 3], [2 2])
      | plot([0 3], [-2 -2])
      | color('black')
      | 
      | plot([0 2 2 3], [1 1 0 0])
      | plot([1 3 2 1 0 2], [0.6 0.6 0.4 0.6 0.4 0.4])
      | patch([1 3 2],[0.6 0.6 0.4],[0,0,0])
      | plot([0 1 1], [1 1 0.6])
      | plot([1 1 0], [0.4 -1 -1])
  Simplex : Subsystem  Tag=Electrical  Commented=on  InitFcn=initSimplex
      mask Display:
      | color('white')
      | plot([0 3], [2 2])
      | plot([0 3], [-2 -2])
      | color('black')
      | 
      | plot([0 2 2 3], [1 1 0 0])
      | plot([1 3 2 1 0 2], [0.6 0.6 0.4 0.6 0.4 0.4])
      | patch([1 3 2],[0.6 0.6 0.4],[0,0,0])
      | plot([0 1 1], [1 1 0.6])
      | plot([1 1 0], [0.4 -1 -1])
  SimplexSav : Subsystem  Commented=on  InitFcn=initSimplex
      mask Display:
      | plot([0 2 2 3], [1 1 0 0])
      | plot([1 3 2 1 0 2], [0.6 0.6 0.4 0.6 0.4 0.4])
      | patch([1 3 2],[0.6 0.6 0.4],[0,0,0])
      | plot([0 1 1], [1 1 0.6])
      | plot([1 1 0], [0.4 -1 -1])
      | 
      | color('white')
      | plot([0 3], [2 2])
      | plot([0 3], [-2 -2])
  wires:
  Inflow_old/1(out) -> Inflow_old1/1(in)
  Inflow_old1/1(out) -> Outflow_old1/1(in)
  Outflow_old1/1(out) -> Mux/1
  Outflow_old1/2(backs) -> Inflow_old1/2(back), Mux/2

== system Simple_lib/Driveline/Brake ==
  ctrl : Inport
  in : Inport  Port=2
  T : Inport  Port=3
  Friction : $bdroot/Rotational/Friction  grab=1  s=1  Ki=100
  Ground1 : Ground
  Terminator1 : Terminator
  Terminator2 : Terminator
  _out1 : $bdroot/Rotational/_out  Tag=Electrical  Level=v  Flow=F
  wires:
  in/1 -> Friction/3
  ctrl/1 -> Friction/2
  T/1 -> Terminator1/1
  _out1/1 -> Friction/1
  _out1/2 -> Terminator2/1  "N"
  Ground1/1 -> _out1/1
